simulink model "ext_steer_col_gear"  (Simulink 8.2)
settings: Solver=ode45  SolverMode=SingleTasking  StartTime=0  StopTime=110  FixedStep=0.002  RelTol=1e-3  AbsTol=1e-6
libraries: Solver_SF x1, simulink_extras x1
settings Model: Creator=ywata  LastModifiedBy=dhall  ExtModeTrigMode=oneshot  ExtModeArmWhenConnect=off
settings DataIOCC: LimitDataPoints=off  SignalLoggingName=sigsOut
settings OptimizationCC: BlockReduction=off  BooleanDataType=off  ExpressionDepthLimit=128
settings DebuggingCC: SaveWithParameterizedLinksMsg=none  SignalResolutionControl=TryResolveAllWithWarning  SolverPrmCheckMsg=none  MultiTaskDSMMsg=warning  MultiTaskCondExecSysMsg=none
settings HardwareCC: TargetUnknown=on
settings RTWCC: TemplateMakefile=grt_vc.tmf  IncludeERTFirstTime=on
settings GRTTargetCC: TargetFcnLib=ansi_tfl_tmw.mat

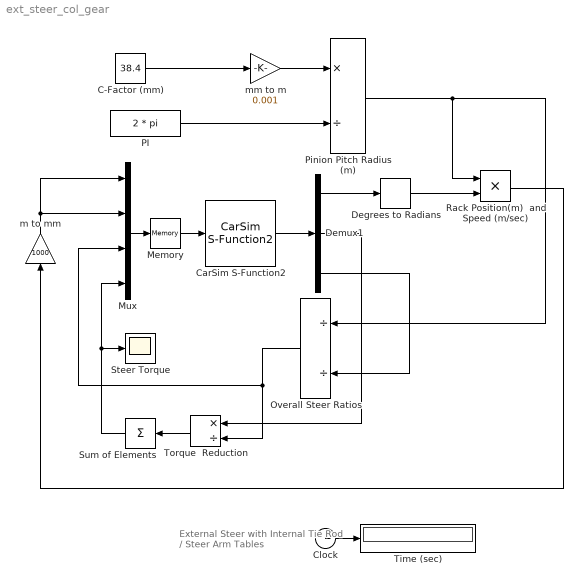
== system ext_steer_col_gear ==
  note: External Steer with Internal
      | Tie Rod / Steer Arm Tables
  C-Factor (mm) : Constant  Value=38.4
  CarSim S-Function2 : Solver_SF/CarSim S-Function2  Priority=1  VehicleCode=i_i  SIMFILE=simfile.sim
      settings: AttributesFormatString=Vehicle Code: %<VehicleCode>
  Clock : Clock
  Degrees to Radians : simulink_extras/Transformations/Degrees to Radians
  Demux1 : Demux  Outputs=[2 2 2]
  Memory : Memory
  Mux : Mux  Inputs=[2 2 2 1]
  Overall Steer Ratios : Product  Inputs=//
  PI : Constant  Value=2 * pi
  "Pinion Pitch Radius (m) " : Product  Inputs=*/
  "Rack Position(m)  and Speed (m/sec)  " : Product
  Steer Torque : Scope
      settings: TickLabels=on  TimeRange=7  SampleTime=100
  Sum of Elements : Sum  Inputs=+
  Time (sec) : Display
      settings: Format=bank  Decimation=100
  Torque  Reduction : Product  Inputs=*/
  m to mm : Gain  Gain=1000
  mm to m : Gain  Gain=0.001
  wires:
  Clock/1 -> Time (sec)/1
  C-Factor (mm)/1 -> mm to m/1
  PI/1 -> "Pinion Pitch Radius (m) "/2
  "Pinion Pitch Radius (m) "/1 -> Overall Steer Ratios/1, "Rack Position(m)  and Speed (m/sec)  "/1
  Overall Steer Ratios/1 -> Torque  Reduction/2, Mux/3
  "Rack Position(m)  and Speed (m/sec)  "/1 -> m to mm/1
  Sum of Elements/1 -> Steer Torque/1, Mux/4
  Demux1/1 -> Degrees to Radians/1
  Degrees to Radians/1 -> "Rack Position(m)  and Speed (m/sec)  "/2
  mm to m/1 -> "Pinion Pitch Radius (m) "/1
  Demux1/3 -> Overall Steer Ratios/2
  Torque  Reduction/1 -> Sum of Elements/1
  m to mm/1 -> Mux/1, Mux/2
  Demux1/2 -> Torque  Reduction/1
  CarSim S-Function2/1 -> Demux1/1
  Mux/1 -> Memory/1
  Memory/1 -> CarSim S-Function2/1
